simulink model "vrmaglev"  (R2016b)
settings: Solver=ode5  StartTime=0.0  StopTime=5  FixedStep=1e-3  MaxStep=0.001  RelTol=1e-3  AbsTol=1e-5
model workspace (MATLAB code in the model file):
  | Ts=1e-3;
undefined symbols (not defined in the file): Gc, Gd_tustin_T2, Gdb, Kdd, Kid, Kpd, m, N1, yd
libraries: simulink x5
Description:
  | Magnetic Levitation Model
  | 
  | vrmaglev is an example showing the interaction between dynamic models in Simulink(R)
  | and virtual worlds. The Simulink model represents the HUMUSOFT(R) CE152 Magnetic Levitation
  | educational / presentation scale model. (http://www.humusoft.com/link/models)
  | 
  | The plant model is controlled by a PID controller with feed forward to cope with the nonlinearity
  | of the magnetic levitation system.
  | 
  | The position of the ball responds to the changing value of the setpoint. You can observe
  | this change not only in the Scope window, but also in a viewer window displaying
  | the virtual world. Note that the position of the ball represents the real dynamics of the system.
  | If you switch the VRML viewer to the Camera 3 viewpoint, you can observe and control the ball easier.
  | 
  | There are two possible methods of setting the ball position setpoint - using a Signal Generator
  | and visually by clicking at a desired position in the virtual reality scene.
  | 
  | In the virtual scene, a VRML sensor is defined. If you click in the space between the magnetic coil
  | and the bottom plate, VRML sensor is updated and its value is read into Simulink model using the
  | VR Source block.
settings Model: FPTRunName=Active  ExtModeTrigDuration=5000  ExtModeTrigLevel=0.500000  Creator=The MathWorks, Inc.  LastModifiedBy=nimaz
settings DataIOCC: SaveFormat=Array  SaveOutput=off  SaveTime=off  SignalLoggingName=logsOut
settings OptimizationCC: BlockReduction=off  BooleanDataType=off  OptimizeBlockIOStorage=off  BufferReuse=off  GlobalBufferReuse=off  ExpressionFolding=off  ExpressionDepthLimit=2147483647  LocalBlockOutputs=off  InitFltsAndDblsToZero=on  LifeSpan=inf
settings DebuggingCC: UnderspecifiedInitializationDetection=Classic  MergeDetectMultiDrivingBlocksExec=none  CheckExecutionContextPreStartOutputMsg=on  SignalResolutionControl=TryResolveAllWithWarning  MultiTaskDSMMsg=warning  MultiTaskCondExecSysMsg=none  FcnCallInpInsideContextMsg=warning  StateNameClashWarn=warning  SFUnexpectedBacktrackingDiag=warning  SFNoUnconditionalDefaultTransitionDiag=warning  SFExecutionAtInitializationDiag=none
settings HardwareCC: ProdBitPerPointer=32  ProdBitPerSizeT=32  ProdBitPerPtrDiffT=32  ProdLargestAtomicFloat=None  ProdIntDivRoundTo=Undefined  ProdEndianess=Unspecified  ProdWordSize=32  ProdHWDeviceType=32-bit Generic  TargetUnknown=on
settings ModelReferenceCC: UpdateModelReferenceTargets=IfOutOfDate  PropagateSignalLabelsOutOfModel=off
settings RTWCC: RetainRTWFile=on
settings GRTTargetCC: TargetFcnLib=ansi_tfl_tmw.mat  TargetLangStandard=C89/C90 (ANSI)  CombineOutputUpdateFcns=off  GRTInterface=on
settings ConfigComp: CovMetricSettings=d  CovSaveCumulativeToWorkspaceVar=on  CovSaveSingleToWorkspaceVar=on  CovExternalEMLEnable=off  CovSFcnEnable=off

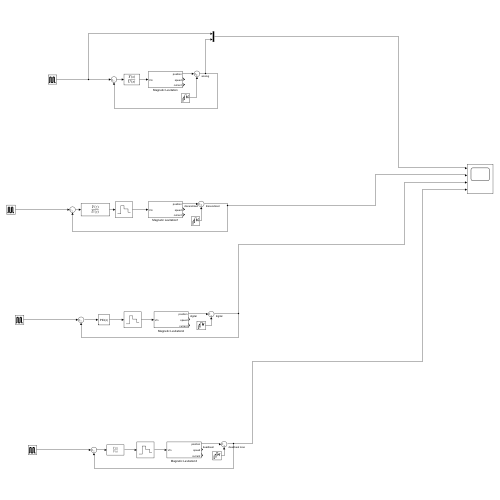
[thumbnail: Simulink's stored preview of the top-level diagram]
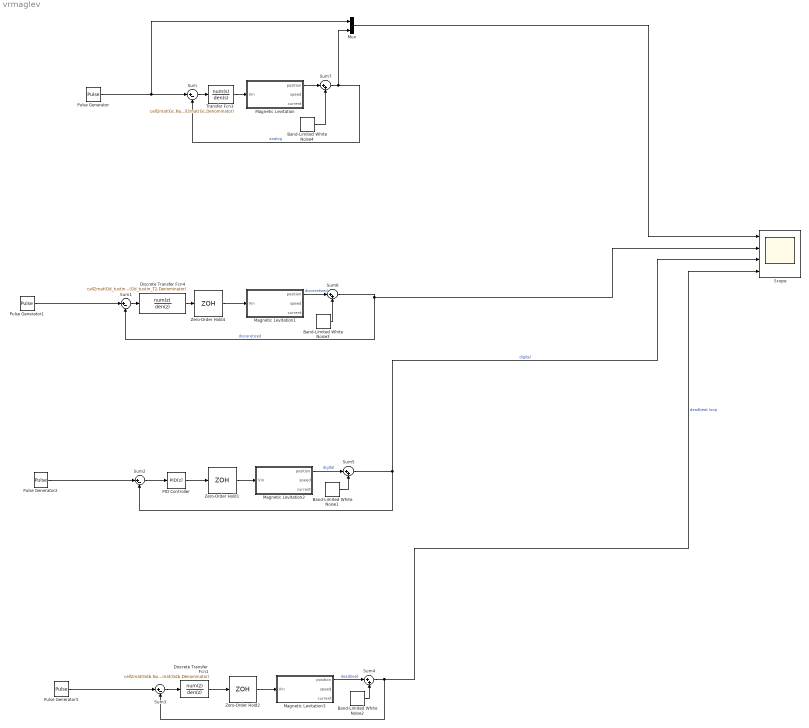
== system vrmaglev ==
  Band-Limited White Noise{1..4} (4 alike) : simulink/Sources/Band-Limited White Noise  Cov=1e-5  Ts=0.01  seed=[23341]
  Discrete Transfer Fcn1 : DiscreteTransferFcn  Numerator=cell2mat(Gdb.Numerator)  Denominator=cell2mat(Gdb.Denominator)  SampleTime=0.01
  Discrete Transfer Fcn4 : DiscreteTransferFcn  Numerator=cell2mat(Gd_tustin_T2.Numerator)  Denominator=cell2mat(Gd_tustin_T2.Denominator)  SampleTime=0.01
  Magnetic Levitation : Subsystem
  Magnetic Levitation1 : Subsystem
  Magnetic Levitation2 : Subsystem
  Magnetic Levitation3 : Subsystem
  Mux : Mux  Inputs=2
  PID Controller : simulink/Continuous/PID Controller  Controller=PID  Form=Parallel  TimeDomain=Discrete-time  SampleTime=0.01  IntegratorMethod=Forward Euler  ControllerParametersSource=internal  P=Kpd  I=Kid  D=Kdd  N=N1  UseFilter=on  InitialConditionSource=internal  InitialConditionForIntegrator=0  InitialConditionForFilter=0  DifferentiatorICPrevScaledInput=0  ExternalReset=none  TrackingMode=off  Kt=1  LimitOutput=off  UpperSaturationLimit=inf  LowerSaturationLimit=-inf  LinearizeAsGain=on  AntiWindupMode=none  Kb=1  POutMin=[]  POutMax=[]  IOutMin=[]  IOutMax=[]  DOutMin=[]  DOutMax=[]  NOutMin=[]  NOutMax=[]  SumOutMin=[]  SumOutMax=[]  SaturationOutMin=[]  SaturationOutMax=[]  PParamMin=[]  PParamMax=[]  IParamMin=[]  IParamMax=[]  DParamMin=[]  DParamMax=[]  NParamMin=[]  NParamMax=[]  KbParamMin=[]  KbParamMax=[]  KtParamMin=[]  KtParamMax=[]  KbOutMin=[]  KbOutMax=[]  KtOutMin=[]  KtOutMax=[]  IntegratorOutMin=[]  IntegratorOutMax=[]  FilterOutMin=[]  FilterOutMax=[]  SumI1OutMin=[]  SumI1OutMax=[]  SumI2OutMin=[]  SumI2OutMax=[]  SumI3OutMin=[]  SumI3OutMax=[]  SumDOutMin=[]  SumDOutMax=[]  DifferentiatorOutMin=[]  DifferentiatorOutMax=[]  IntegratorContinuousStateAttributes=''  IntegratorStateMustResolveToSignalObject=off  IntegratorRTWStateStorageClass=Auto  FilterContinuousStateAttributes=''  FilterStateMustResolveToSignalObject=off  FilterRTWStateStorageClass=Auto
  Pulse Generator{,1..3} (4 alike) : DiscretePulseGenerator  PulseType=Time based  Amplitude=yd  Period=11  PulseWidth=50
  Scope : Scope  NumInputPorts=4
  Sum{,1..3} (4 alike) : Sum  Inputs=|+-  InputSameDT=on  SaturateOnIntegerOverflow=on  OutDataTypeStr=Inherit: Same as first input
  Sum{4..7} (4 alike) : Sum  Inputs=|++
  Transfer Fcn3 : TransferFcn  Numerator=cell2mat(Gc.Numerator)  Denominator=cell2mat(Gc.Denominator)
  Zero-Order Hold1 : ZeroOrderHold  SampleTime=0.01
  Zero-Order Hold2 : ZeroOrderHold  SampleTime=0.01
  Zero-Order Hold4 : ZeroOrderHold  SampleTime=0.01
  wires:
  Mux/1 -> Scope/1
  Pulse Generator/1 -> Mux/1, Sum/1
  Sum/1 -> Transfer Fcn3/1
  Transfer Fcn3/1 -> Magnetic Levitation/1(Vin)
  Pulse Generator1/1 -> Sum1/1
  Sum1/1 -> Discrete Transfer Fcn4/1
  Discrete Transfer Fcn4/1 -> Zero-Order Hold4/1
  Zero-Order Hold4/1 -> Magnetic Levitation1/1(Vin)
  Zero-Order Hold1/1 -> Magnetic Levitation2/1(Vin)
  Sum2/1 -> PID Controller/1
  PID Controller/1 -> Zero-Order Hold1/1
  Pulse Generator2/1 -> Sum2/1
  Zero-Order Hold2/1 -> Magnetic Levitation3/1(Vin)
  Discrete Transfer Fcn1/1 -> Zero-Order Hold2/1
  Sum3/1 -> Discrete Transfer Fcn1/1
  Pulse Generator3/1 -> Sum3/1
  Band-Limited White Noise2/1 -> Sum4/2
  Sum4/1 -> Scope/4, Sum3/2  "deadbeat loop"
  Magnetic Levitation3/1(position) -> Sum4/1  "deadbeat"
  Band-Limited White Noise1/1 -> Sum5/2
  Magnetic Levitation2/1(position) -> Sum5/1  "digital"
  Sum5/1 -> Scope/3, Sum2/2  "digital"
  Band-Limited White Noise3/1 -> Sum6/2
  Magnetic Levitation1/1(position) -> Sum6/1  "disceretized"
  Sum6/1 -> Sum1/2, Scope/2  "disceretized"
  Band-Limited White Noise4/1 -> Sum7/2
  Magnetic Levitation/1(position) -> Sum7/1
  Sum7/1 -> Sum/2, Mux/2  "analog"

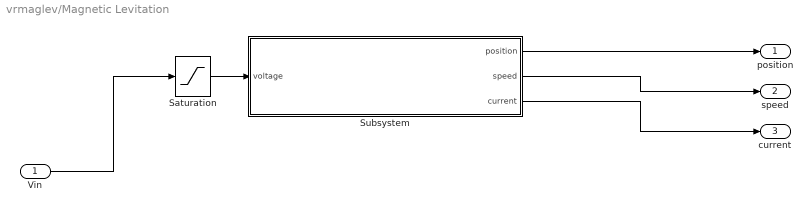
== system vrmaglev/Magnetic Levitation ==
  Vin : Inport
  Saturation : Saturate  UpperLimit=10  LowerLimit=0  ZeroCross=off
  Subsystem : Subsystem
  position : Outport
  speed : Outport  Port=2
  current : Outport  Port=3
  wires:
  Vin/1 -> Saturation/1
  Saturation/1 -> Subsystem/1(voltage)
  Subsystem/1("position ") -> position/1
  Subsystem/2(speed) -> speed/1
  Subsystem/3(current) -> current/1

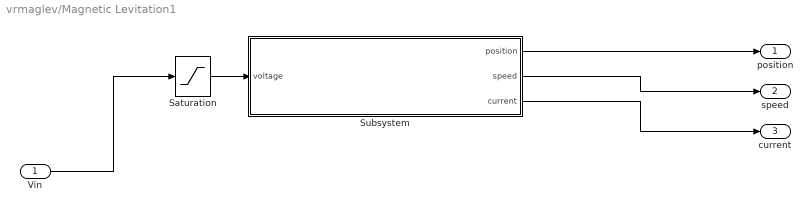
== system vrmaglev/Magnetic Levitation1 ==
  Vin : Inport
  Saturation : Saturate  UpperLimit=10  LowerLimit=0  ZeroCross=off
  Subsystem : Subsystem
  position : Outport
  speed : Outport  Port=2
  current : Outport  Port=3
  wires:
  Vin/1 -> Saturation/1
  Saturation/1 -> Subsystem/1(voltage)
  Subsystem/1("position ") -> position/1
  Subsystem/2(speed) -> speed/1
  Subsystem/3(current) -> current/1

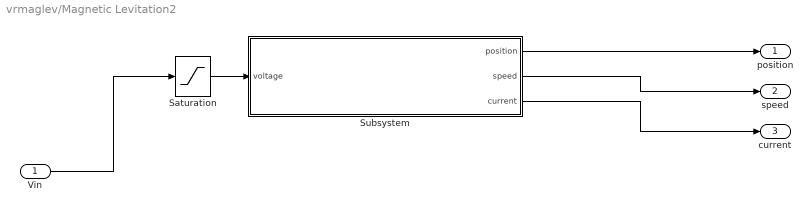
== system vrmaglev/Magnetic Levitation2 ==
  Vin : Inport
  Saturation : Saturate  UpperLimit=10  LowerLimit=0  ZeroCross=off
  Subsystem : Subsystem
  position : Outport
  speed : Outport  Port=2
  current : Outport  Port=3
  wires:
  Vin/1 -> Saturation/1
  Saturation/1 -> Subsystem/1(voltage)
  Subsystem/1("position ") -> position/1
  Subsystem/2(speed) -> speed/1
  Subsystem/3(current) -> current/1

== system vrmaglev/Magnetic Levitation3 ==
  Vin : Inport
  Saturation : Saturate  UpperLimit=10  LowerLimit=0  ZeroCross=off
  Subsystem : Subsystem
  position : Outport
  speed : Outport  Port=2
  current : Outport  Port=3
  wires:
  Vin/1 -> Saturation/1
  Saturation/1 -> Subsystem/1(voltage)
  Subsystem/1("position ") -> position/1
  Subsystem/2(speed) -> speed/1
  Subsystem/3(current) -> current/1

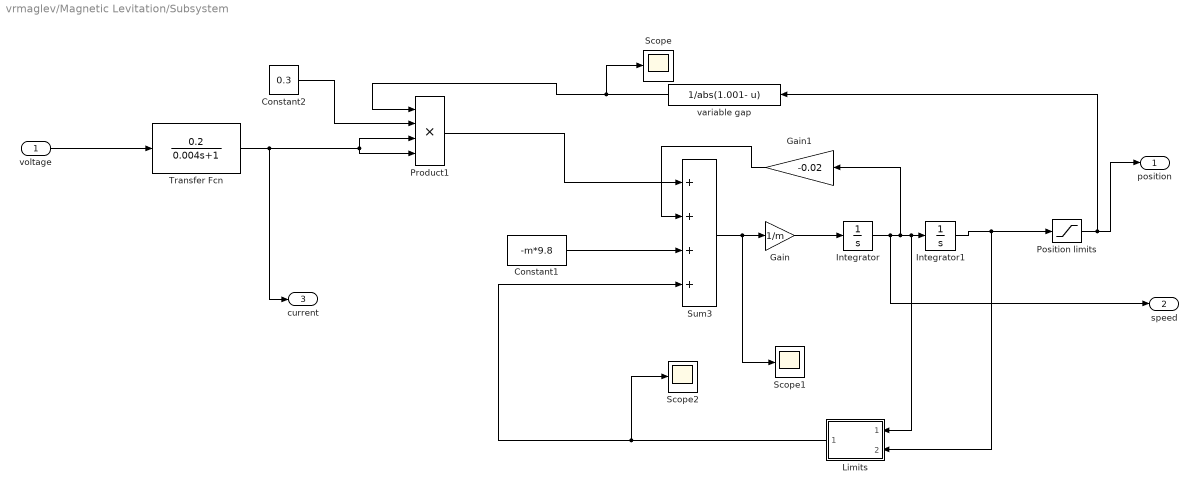
== system vrmaglev/Magnetic Levitation/Subsystem ==
  voltage : Inport
  Constant1 : Constant  Value=-m*9.8
  Constant2 : Constant  Value=0.3
  Gain : Gain  Gain=1/m
  Gain1 : Gain  Gain=-0.02
  Integrator : Integrator
  Integrator1 : Integrator  LimitOutput=on  UpperSaturationLimit=1  LowerSaturationLimit=0
  Limits : Subsystem
      mask Display: disp('LIMIT')
  Position limits : Saturate  UpperLimit=0.998  LowerLimit=0.001  ZeroCross=off
  Product1 : Product  Inputs=4
  Scope : Scope
  Scope1 : Scope
  Scope2 : Scope
  Sum3 : Sum  Inputs=++++
  Transfer Fcn : TransferFcn  Numerator=[0.2]  Denominator=[0.004 1]
  variable gap : Fcn  Expr=1/abs(1.001- u)
  "position " : Outport
  speed : Outport  Port=2
  current : Outport  Port=3
  wires:
  Position limits/1 -> variable gap/1, "position "/1
  Integrator1/1 -> Limits/2(position), Position limits/1
  Sum3/1 -> Scope1/1, Gain/1
  Constant2/1 -> Product1/2
  Constant1/1 -> Sum3/3
  variable gap/1 -> Scope/1, Product1/1
  Gain1/1 -> Sum3/2
  Gain/1 -> Integrator/1
  Integrator/1 -> speed/1, Limits/1(velocity), Integrator1/1, Gain1/1
  Product1/1 -> Sum3/1
  Transfer Fcn/1 -> current/1, Product1/3, Product1/4
  voltage/1 -> Transfer Fcn/1
  Limits/1(force) -> Scope2/1, Sum3/4

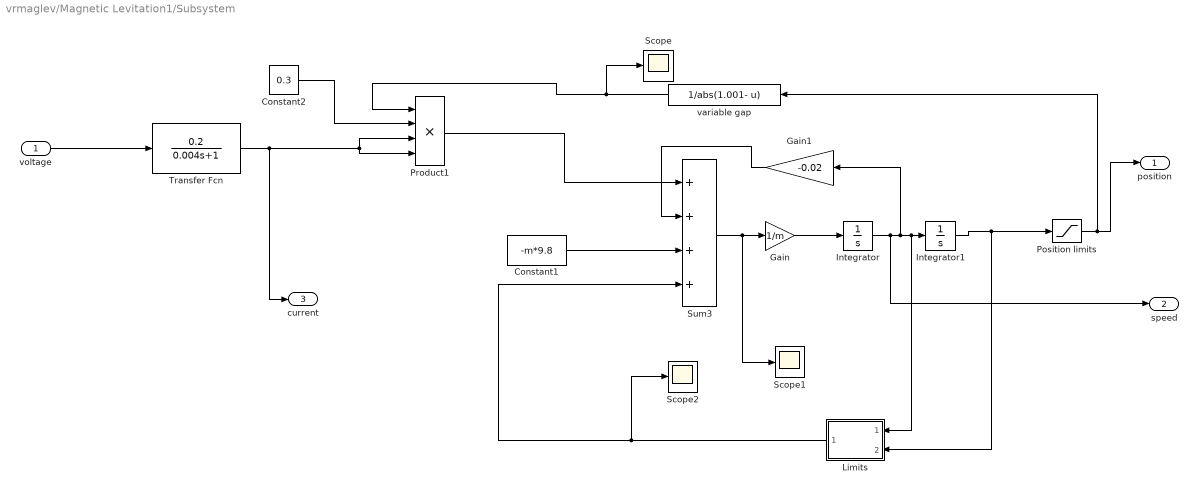
== system vrmaglev/Magnetic Levitation1/Subsystem ==
  voltage : Inport
  Constant1 : Constant  Value=-m*9.8
  Constant2 : Constant  Value=0.3
  Gain : Gain  Gain=1/m
  Gain1 : Gain  Gain=-0.02
  Integrator : Integrator
  Integrator1 : Integrator  LimitOutput=on  UpperSaturationLimit=1  LowerSaturationLimit=0
  Limits : Subsystem
      mask Display: disp('LIMIT')
  Position limits : Saturate  UpperLimit=0.998  LowerLimit=0.001  ZeroCross=off
  Product1 : Product  Inputs=4
  Scope : Scope
  Scope1 : Scope
  Scope2 : Scope
  Sum3 : Sum  Inputs=++++
  Transfer Fcn : TransferFcn  Numerator=[0.2]  Denominator=[0.004 1]
  variable gap : Fcn  Expr=1/abs(1.001- u)
  "position " : Outport
  speed : Outport  Port=2
  current : Outport  Port=3
  wires:
  Position limits/1 -> variable gap/1, "position "/1
  Integrator1/1 -> Limits/2(position), Position limits/1
  Sum3/1 -> Scope1/1, Gain/1
  Constant2/1 -> Product1/2
  Constant1/1 -> Sum3/3
  variable gap/1 -> Scope/1, Product1/1
  Gain1/1 -> Sum3/2
  Gain/1 -> Integrator/1
  Integrator/1 -> speed/1, Limits/1(velocity), Integrator1/1, Gain1/1
  Product1/1 -> Sum3/1
  Transfer Fcn/1 -> current/1, Product1/3, Product1/4
  voltage/1 -> Transfer Fcn/1
  Limits/1(force) -> Scope2/1, Sum3/4

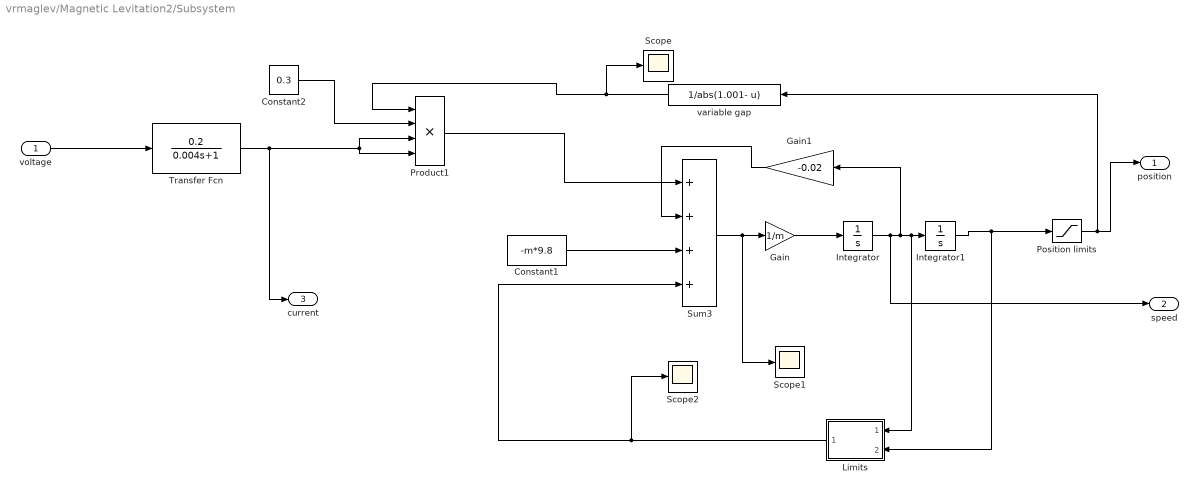
== system vrmaglev/Magnetic Levitation2/Subsystem ==
  voltage : Inport
  Constant1 : Constant  Value=-m*9.8
  Constant2 : Constant  Value=0.3
  Gain : Gain  Gain=1/m
  Gain1 : Gain  Gain=-0.02
  Integrator : Integrator
  Integrator1 : Integrator  LimitOutput=on  UpperSaturationLimit=1  LowerSaturationLimit=0
  Limits : Subsystem
      mask Display: disp('LIMIT')
  Position limits : Saturate  UpperLimit=0.998  LowerLimit=0.001  ZeroCross=off
  Product1 : Product  Inputs=4
  Scope : Scope
  Scope1 : Scope
  Scope2 : Scope
  Sum3 : Sum  Inputs=++++
  Transfer Fcn : TransferFcn  Numerator=[0.2]  Denominator=[0.004 1]
  variable gap : Fcn  Expr=1/abs(1.001- u)
  "position " : Outport
  speed : Outport  Port=2
  current : Outport  Port=3
  wires:
  Position limits/1 -> variable gap/1, "position "/1
  Integrator1/1 -> Limits/2(position), Position limits/1
  Sum3/1 -> Scope1/1, Gain/1
  Constant2/1 -> Product1/2
  Constant1/1 -> Sum3/3
  variable gap/1 -> Scope/1, Product1/1
  Gain1/1 -> Sum3/2
  Gain/1 -> Integrator/1
  Integrator/1 -> speed/1, Limits/1(velocity), Integrator1/1, Gain1/1
  Product1/1 -> Sum3/1
  Transfer Fcn/1 -> current/1, Product1/3, Product1/4
  voltage/1 -> Transfer Fcn/1
  Limits/1(force) -> Scope2/1, Sum3/4

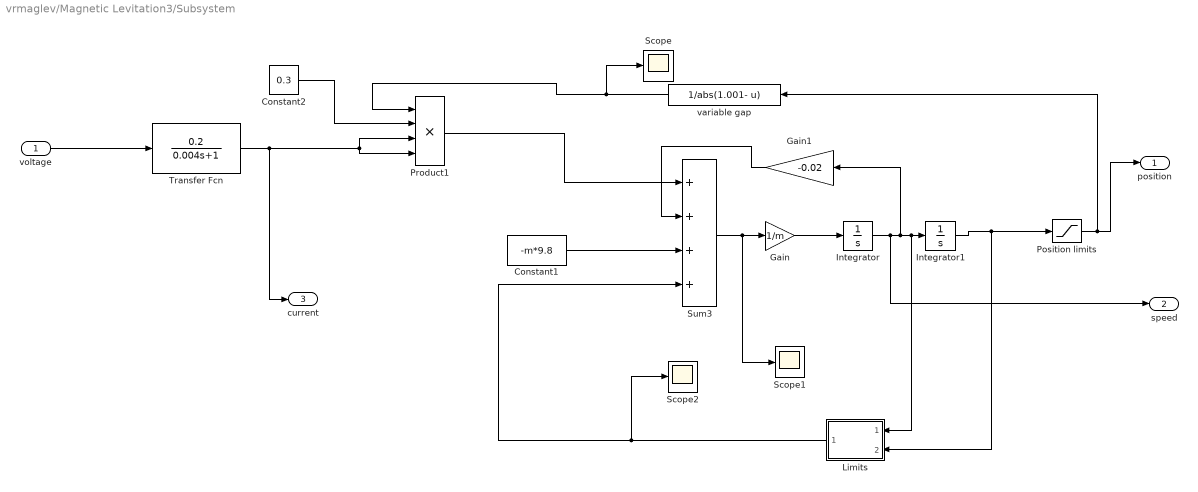
== system vrmaglev/Magnetic Levitation3/Subsystem ==
  voltage : Inport
  Constant1 : Constant  Value=-m*9.8
  Constant2 : Constant  Value=0.3
  Gain : Gain  Gain=1/m
  Gain1 : Gain  Gain=-0.02
  Integrator : Integrator
  Integrator1 : Integrator  LimitOutput=on  UpperSaturationLimit=1  LowerSaturationLimit=0
  Limits : Subsystem
      mask Display: disp('LIMIT')
  Position limits : Saturate  UpperLimit=0.998  LowerLimit=0.001  ZeroCross=off
  Product1 : Product  Inputs=4
  Scope : Scope
  Scope1 : Scope
  Scope2 : Scope
  Sum3 : Sum  Inputs=++++
  Transfer Fcn : TransferFcn  Numerator=[0.2]  Denominator=[0.004 1]
  variable gap : Fcn  Expr=1/abs(1.001- u)
  "position " : Outport
  speed : Outport  Port=2
  current : Outport  Port=3
  wires:
  Position limits/1 -> variable gap/1, "position "/1
  Integrator1/1 -> Limits/2(position), Position limits/1
  Sum3/1 -> Scope1/1, Gain/1
  Constant2/1 -> Product1/2
  Constant1/1 -> Sum3/3
  variable gap/1 -> Scope/1, Product1/1
  Gain1/1 -> Sum3/2
  Gain/1 -> Integrator/1
  Integrator/1 -> speed/1, Limits/1(velocity), Integrator1/1, Gain1/1
  Product1/1 -> Sum3/1
  Transfer Fcn/1 -> current/1, Product1/3, Product1/4
  voltage/1 -> Transfer Fcn/1
  Limits/1(force) -> Scope2/1, Sum3/4

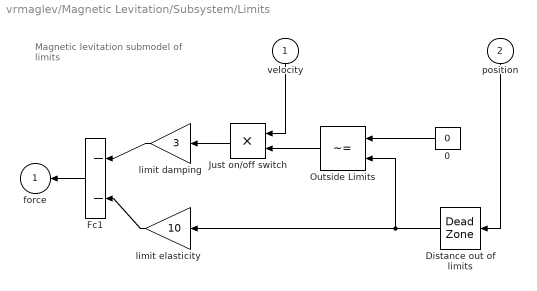
== system vrmaglev/Magnetic Levitation/Subsystem/Limits ==
  note: Magnetic levitation
      | submodel of limits
  velocity : Inport
  position : Inport  Port=2
  0 : Constant  Value=0
  Distance out of limits : DeadZone  LowerValue=0.002  UpperValue=1  ZeroCross=off  SaturateOnIntegerOverflow=on
  Fc1 : Sum  Inputs=--  InputSameDT=on  SaturateOnIntegerOverflow=on  OutDataTypeStr=Inherit: Same as first input
  "Just on/off switch " : Product  InputSameDT=on  SaturateOnIntegerOverflow=on  OutDataTypeStr=Inherit: Same as first input
  Outside Limits : RelationalOperator  Operator=~=  RndMeth=Nearest  InputSameDT=on
  limit damping : Gain  Gain=3  SaturateOnIntegerOverflow=on  OutDataTypeStr=Inherit: Same as input  ParamDataTypeStr=Inherit: Same as input
  limit elasticity : Gain  Gain=10  SaturateOnIntegerOverflow=on  OutDataTypeStr=Inherit: Same as input  ParamDataTypeStr=Inherit: Same as input
  force : Outport
  wires:
  Distance out of limits/1 -> Outside Limits/2, limit elasticity/1
  limit damping/1 -> Fc1/1
  limit elasticity/1 -> Fc1/2
  Outside Limits/1 -> "Just on/off switch "/2
  0/1 -> Outside Limits/1
  "Just on/off switch "/1 -> limit damping/1
  velocity/1 -> "Just on/off switch "/1
  Fc1/1 -> force/1
  position/1 -> Distance out of limits/1

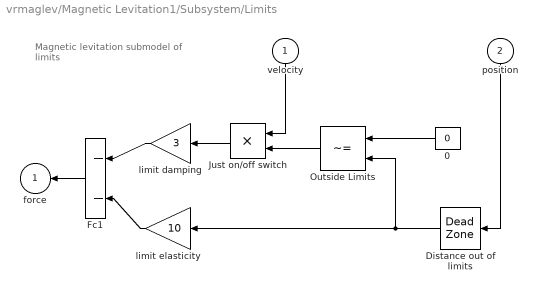
== system vrmaglev/Magnetic Levitation1/Subsystem/Limits ==
  note: Magnetic levitation
      | submodel of limits
  velocity : Inport
  position : Inport  Port=2
  0 : Constant  Value=0
  Distance out of limits : DeadZone  LowerValue=0.002  UpperValue=1  ZeroCross=off  SaturateOnIntegerOverflow=on
  Fc1 : Sum  Inputs=--  InputSameDT=on  SaturateOnIntegerOverflow=on  OutDataTypeStr=Inherit: Same as first input
  "Just on/off switch " : Product  InputSameDT=on  SaturateOnIntegerOverflow=on  OutDataTypeStr=Inherit: Same as first input
  Outside Limits : RelationalOperator  Operator=~=  RndMeth=Nearest  InputSameDT=on
  limit damping : Gain  Gain=3  SaturateOnIntegerOverflow=on  OutDataTypeStr=Inherit: Same as input  ParamDataTypeStr=Inherit: Same as input
  limit elasticity : Gain  Gain=10  SaturateOnIntegerOverflow=on  OutDataTypeStr=Inherit: Same as input  ParamDataTypeStr=Inherit: Same as input
  force : Outport
  wires:
  Distance out of limits/1 -> Outside Limits/2, limit elasticity/1
  limit damping/1 -> Fc1/1
  limit elasticity/1 -> Fc1/2
  Outside Limits/1 -> "Just on/off switch "/2
  0/1 -> Outside Limits/1
  "Just on/off switch "/1 -> limit damping/1
  velocity/1 -> "Just on/off switch "/1
  Fc1/1 -> force/1
  position/1 -> Distance out of limits/1

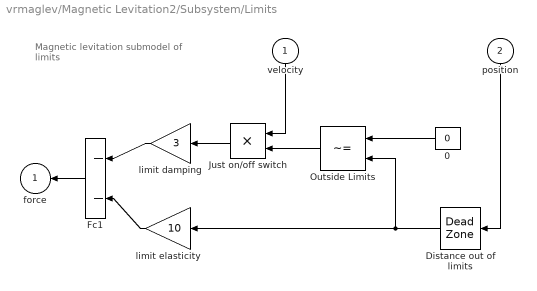
== system vrmaglev/Magnetic Levitation2/Subsystem/Limits ==
  note: Magnetic levitation
      | submodel of limits
  velocity : Inport
  position : Inport  Port=2
  0 : Constant  Value=0
  Distance out of limits : DeadZone  LowerValue=0.002  UpperValue=1  ZeroCross=off  SaturateOnIntegerOverflow=on
  Fc1 : Sum  Inputs=--  InputSameDT=on  SaturateOnIntegerOverflow=on  OutDataTypeStr=Inherit: Same as first input
  "Just on/off switch " : Product  InputSameDT=on  SaturateOnIntegerOverflow=on  OutDataTypeStr=Inherit: Same as first input
  Outside Limits : RelationalOperator  Operator=~=  RndMeth=Nearest  InputSameDT=on
  limit damping : Gain  Gain=3  SaturateOnIntegerOverflow=on  OutDataTypeStr=Inherit: Same as input  ParamDataTypeStr=Inherit: Same as input
  limit elasticity : Gain  Gain=10  SaturateOnIntegerOverflow=on  OutDataTypeStr=Inherit: Same as input  ParamDataTypeStr=Inherit: Same as input
  force : Outport
  wires:
  Distance out of limits/1 -> Outside Limits/2, limit elasticity/1
  limit damping/1 -> Fc1/1
  limit elasticity/1 -> Fc1/2
  Outside Limits/1 -> "Just on/off switch "/2
  0/1 -> Outside Limits/1
  "Just on/off switch "/1 -> limit damping/1
  velocity/1 -> "Just on/off switch "/1
  Fc1/1 -> force/1
  position/1 -> Distance out of limits/1

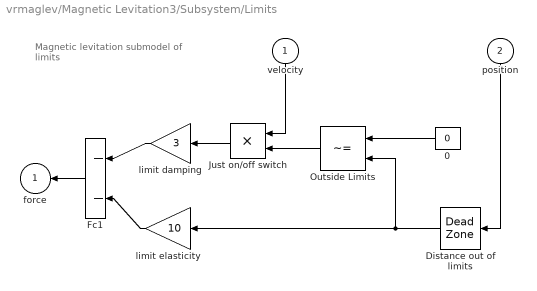
== system vrmaglev/Magnetic Levitation3/Subsystem/Limits ==
  note: Magnetic levitation
      | submodel of limits
  velocity : Inport
  position : Inport  Port=2
  0 : Constant  Value=0
  Distance out of limits : DeadZone  LowerValue=0.002  UpperValue=1  ZeroCross=off  SaturateOnIntegerOverflow=on
  Fc1 : Sum  Inputs=--  InputSameDT=on  SaturateOnIntegerOverflow=on  OutDataTypeStr=Inherit: Same as first input
  "Just on/off switch " : Product  InputSameDT=on  SaturateOnIntegerOverflow=on  OutDataTypeStr=Inherit: Same as first input
  Outside Limits : RelationalOperator  Operator=~=  RndMeth=Nearest  InputSameDT=on
  limit damping : Gain  Gain=3  SaturateOnIntegerOverflow=on  OutDataTypeStr=Inherit: Same as input  ParamDataTypeStr=Inherit: Same as input
  limit elasticity : Gain  Gain=10  SaturateOnIntegerOverflow=on  OutDataTypeStr=Inherit: Same as input  ParamDataTypeStr=Inherit: Same as input
  force : Outport
  wires:
  Distance out of limits/1 -> Outside Limits/2, limit elasticity/1
  limit damping/1 -> Fc1/1
  limit elasticity/1 -> Fc1/2
  Outside Limits/1 -> "Just on/off switch "/2
  0/1 -> Outside Limits/1
  "Just on/off switch "/1 -> limit damping/1
  velocity/1 -> "Just on/off switch "/1
  Fc1/1 -> force/1
  position/1 -> Distance out of limits/1
